simulink model "ageValid_block_unit_test"  (R2018a)
settings: Solver=VariableStepAuto  StartTime=0.0  StopTime=50  RelTol=1e-3
libraries: LeafEcoTronDBWLib x1
settings Model: Creator=TianhuaZhang  LastModifiedBy=TianhuaZhang

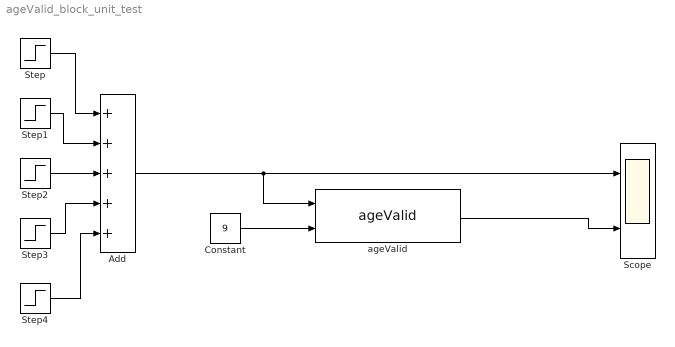
== system ageValid_block_unit_test ==
  Add : Sum  Inputs=+++++
  Constant : Constant  Value=9
  Scope : Scope  NumInputPorts=2
  Step : Step  SampleTime=0
  Step1 : Step  Time=11  SampleTime=0
  Step2 : Step  Time=21  SampleTime=0
  Step3 : Step  Time=31  SampleTime=0
  Step4 : Step  Time=40  SampleTime=0
  ageValid : LeafEcoTronDBWLib/ageValid
  wires:
  Constant/1 -> ageValid/2
  ageValid/1 -> Scope/2
  Step/1 -> Add/1
  Step1/1 -> Add/2
  Step2/1 -> Add/3
  Step3/1 -> Add/4
  Step4/1 -> Add/5
  Add/1 -> ageValid/1, Scope/1
